simulink library "lat_dyn_haul_00"  (R2025a)
settings: Solver=VariableStepAuto  StartTime=0.0  StopTime=10.0  RelTol=1e-3
undefined symbols (not defined in the file): Cf, Cr, Lf, Lr, Machine_Mass, Payload
settings Model: Creator=marti343  LastModifiedBy=marti343

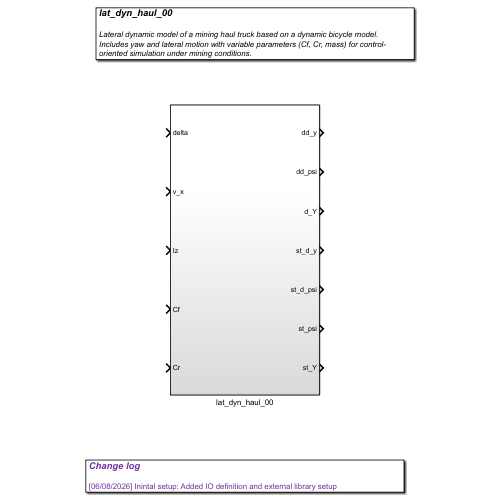
[thumbnail: Simulink's stored preview of the top-level diagram]
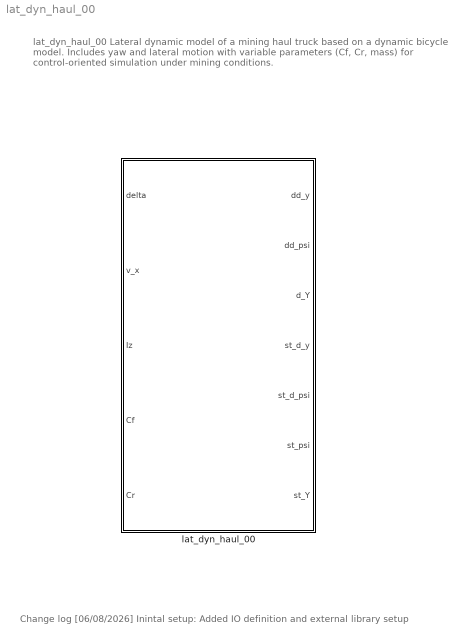
== system lat_dyn_haul_00 ==
  note: lat_dyn_haul_00
      |
      | Lateral dynamic model of a mining haul truck based on a dynamic bicycle model.
      | Includes yaw and lateral motion with variable parameters (Cf, Cr, mass) for control-oriented simulation under mining conditions.
  note: Change log
      |
      | [06/08/2026] Inintal setup: Added IO definition and external library setup
  lat_dyn_haul_00 : Subsystem

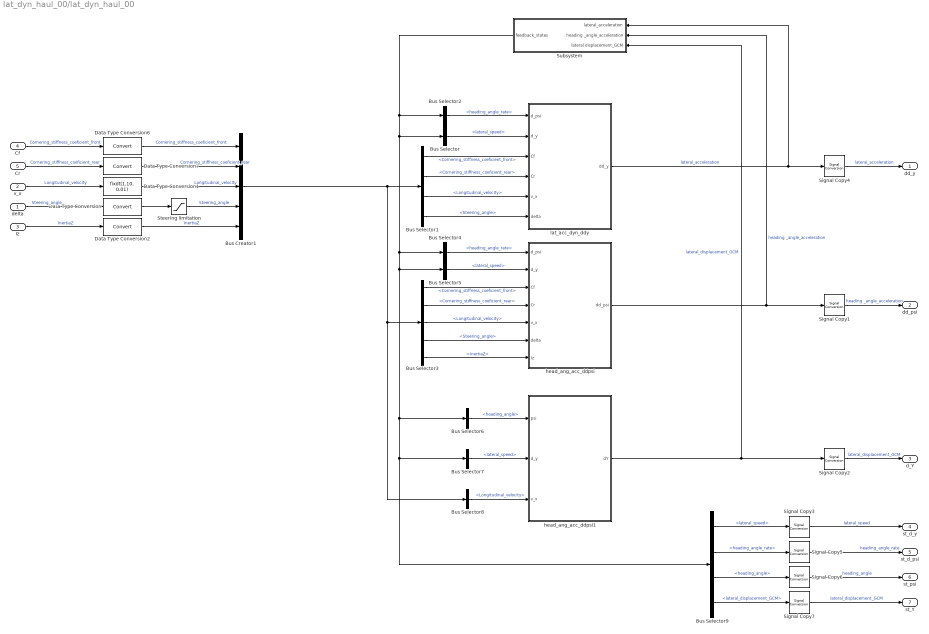
== system lat_dyn_haul_00/lat_dyn_haul_00 ==
  delta : Inport
  v_x : Inport  Port=2
  Iz : Inport  Port=3
  Cf : Inport  Port=4
  Cr : Inport  Port=5
  Bus Creator1 : BusCreator  Inputs=5
  Bus Selector : BusSelector  OutputSignals=lateral_speed
  Bus Selector1 : BusSelector  OutputSignals=Cornering_stiffness_coeficient_front,Cornering_stiffness_coeficient_rear,Longitudinal_velocity,Steering_angle
  Bus Selector2 : BusSelector  OutputSignals=heading_angle_rate
  Bus Selector3 : BusSelector  OutputSignals=Cornering_stiffness_coeficient_front,Cornering_stiffness_coeficient_rear,Longitudinal_velocity,Steering_angle,InertiaZ
  Bus Selector4 : BusSelector  OutputSignals=heading_angle_rate
  Bus Selector5 : BusSelector  OutputSignals=lateral_speed
  Bus Selector6 : BusSelector  OutputSignals=heading_angle
  Bus Selector7 : BusSelector  OutputSignals=lateral_speed
  Bus Selector8 : BusSelector  OutputSignals=Longitudinal_velocity
  Bus Selector9 : BusSelector  OutputSignals=lateral_speed,heading_angle_rate,heading_angle,lateral_displacement_GCM
  Data Type Conversion{,2,6..7} (4 alike) : DataTypeConversion  SaturateOnIntegerOverflow=off  RndMeth=Floor
  Data Type Conversion1 : DataTypeConversion  OutDataTypeStr=fixdt(1,10, 0.01)  SaturateOnIntegerOverflow=off  RndMeth=Floor
  Signal Copy{1..7} (7 alike) : SignalConversion  OverrideOpt=off
  Steering limitation : Saturate
  Subsystem : Subsystem
  head_ang_acc_ddpsi : Subsystem
  head_ang_acc_ddpsi1 : Subsystem
  lat_acc_dyn_ddy : Subsystem
  dd_y : Outport
  dd_psi : Outport  Port=2
  d_Y : Outport  Port=3
  st_d_y : Outport  Port=4
  st_d_psi : Outport  Port=5
  st_psi : Outport  Port=6
  st_Y : Outport  Port=7
  wires:
  delta/1 -> Data Type Conversion/1  "Steering_angle"
  Cf/1 -> Data Type Conversion6/1  "Cornering_stiffness_coeficient_front"
  Iz/1 -> Data Type Conversion2/1  "InertiaZ"
  v_x/1 -> Data Type Conversion1/1  "Longitudinal_velocity"
  Cr/1 -> Data Type Conversion7/1  "Cornering_stiffness_coeficient_rear"
  Data Type Conversion/1 -> Steering limitation/1
  Data Type Conversion6/1 -> Bus Creator1/1  "Cornering_stiffness_coeficient_front"
  Data Type Conversion7/1 -> Bus Creator1/2  "Cornering_stiffness_coeficient_rear"
  Data Type Conversion1/1 -> Bus Creator1/3  "Longitudinal_velocity"
  Steering limitation/1 -> Bus Creator1/4  "Steering_angle"
  lat_acc_dyn_ddy/1(dd_y) -> Subsystem/1(lateral_acceleration), Signal Copy4/1  "lateral_acceleration"
  Bus Selector/1 -> lat_acc_dyn_ddy/2(d_y)  "<lateral_speed>"
  Data Type Conversion2/1 -> Bus Creator1/5  "InertiaZ"
  Bus Creator1/1 -> Bus Selector8/1, Bus Selector3/1, Bus Selector1/1
  Bus Selector1/1 -> lat_acc_dyn_ddy/3(Cf)  "<Cornering_stiffness_coeficient_front>"
  Bus Selector1/2 -> lat_acc_dyn_ddy/4(Cr)  "<Cornering_stiffness_coeficient_rear>"
  Bus Selector1/3 -> lat_acc_dyn_ddy/5(v_x)  "<Longitudinal_velocity>"
  Bus Selector1/4 -> lat_acc_dyn_ddy/6(delta)  "<Steering_angle>"
  head_ang_acc_ddpsi/1(dd_psi) -> Subsystem/2(heading _angle_acceleration), Signal Copy1/1  "heading _angle_acceleration"
  Bus Selector2/1 -> lat_acc_dyn_ddy/1(d_psi)  "<heading_angle_rate>"
  Bus Selector3/1 -> head_ang_acc_ddpsi/3(Cf)  "<Cornering_stiffness_coeficient_front>"
  Bus Selector3/2 -> head_ang_acc_ddpsi/4(Cr)  "<Cornering_stiffness_coeficient_rear>"
  Bus Selector3/3 -> head_ang_acc_ddpsi/5(v_x)  "<Longitudinal_velocity>"
  Bus Selector3/4 -> head_ang_acc_ddpsi/6(delta)  "<Steering_angle>"
  Bus Selector3/5 -> head_ang_acc_ddpsi/7(Iz)  "<InertiaZ>"
  Bus Selector4/1 -> head_ang_acc_ddpsi/1(d_psi)  "<heading_angle_rate>"
  head_ang_acc_ddpsi1/1(dY) -> Subsystem/3(lateral displacement_GCM), Signal Copy2/1  "lateral_displacement_GCM"
  Bus Selector6/1 -> head_ang_acc_ddpsi1/1(psi)  "<heading_angle>"
  Bus Selector5/1 -> head_ang_acc_ddpsi/2(d_y)  "<lateral_speed>"
  Bus Selector7/1 -> head_ang_acc_ddpsi1/2(d_y)  "<lateral_speed>"
  Bus Selector8/1 -> head_ang_acc_ddpsi1/3(v_x)  "<Longitudinal_velocity>"
  Subsystem/1(feedback_states) -> Bus Selector2/1, Bus Selector9/1, Bus Selector7/1, Bus Selector6/1, Bus Selector5/1, Bus Selector4/1, Bus Selector/1
  Signal Copy4/1 -> dd_y/1  "lateral_acceleration"
  Signal Copy1/1 -> dd_psi/1  "heading _angle_acceleration"
  Signal Copy2/1 -> d_Y/1  "lateral_displacement_GCM"
  Bus Selector9/1 -> Signal Copy3/1  "<lateral_speed>"
  Bus Selector9/2 -> Signal Copy5/1  "<heading_angle_rate>"
  Bus Selector9/3 -> Signal Copy6/1  "<heading_angle>"
  Bus Selector9/4 -> Signal Copy7/1  "<lateral_displacement_GCM>"
  Signal Copy3/1 -> st_d_y/1  "lateral_speed"
  Signal Copy5/1 -> st_d_psi/1  "heading_angle_rate"
  Signal Copy6/1 -> st_psi/1  "heading_angle"
  Signal Copy7/1 -> st_Y/1  "lateral_displacement_GCM"

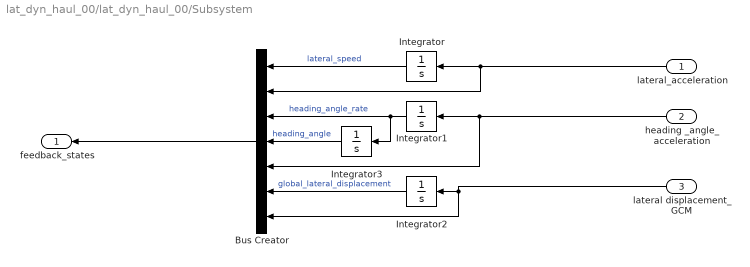
== system lat_dyn_haul_00/lat_dyn_haul_00/Subsystem ==
  lateral_acceleration : Inport
  heading _angle_acceleration : Inport  Port=2
  lateral displacement_GCM : Inport  Port=3
  Bus Creator : BusCreator  Inputs=7
  Integrator : Integrator
  Integrator1 : Integrator  InitialCondition=0.01
  Integrator2 : Integrator
  Integrator3 : Integrator
  feedback_states : Outport
  wires:
  Integrator1/1 -> Integrator3/1, Bus Creator/3  "heading_angle_rate"
  Integrator/1 -> Bus Creator/1  "lateral_speed"
  Integrator2/1 -> Bus Creator/6  "global_lateral_displacement"
  lateral_acceleration/1 -> Integrator/1, Bus Creator/2
  heading _angle_acceleration/1 -> Bus Creator/5, Integrator1/1
  lateral displacement_GCM/1 -> Bus Creator/7, Integrator2/1
  Integrator3/1 -> Bus Creator/4  "heading_angle"
  Bus Creator/1 -> feedback_states/1

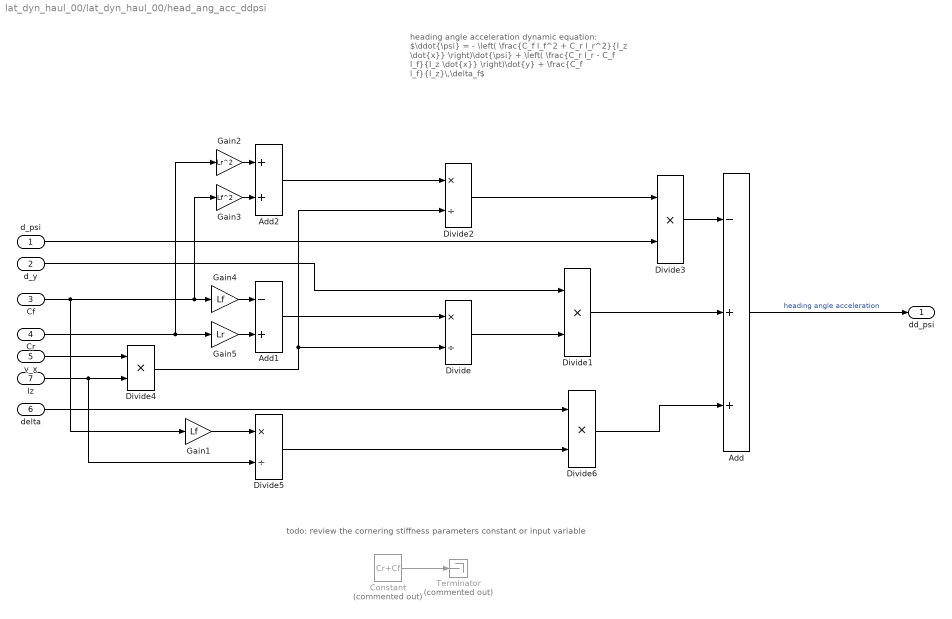
== system lat_dyn_haul_00/lat_dyn_haul_00/head_ang_acc_ddpsi ==
  note: heading angle acceleration dynamic equation:
      |
      | $\ddot{\psi} = - \left( \frac{C_f l_f^2 + C_r l_r^2}{I_z \dot{x}} \right)\dot{\psi} + \left( \frac{C_r l_r - C_f l_f}{I_z \dot{x}} \right)\dot{y} + \frac{C_f l_f}{I_z}\,\delta_f$
  note: todo: review the cornering stiffness parameters constant or input variable
  d_psi : Inport
  d_y : Inport  Port=2
  Cf : Inport  Port=3
  Cr : Inport  Port=4
  v_x : Inport  Port=5
  delta : Inport  Port=6
  Iz : Inport  Port=7
  Add : Sum  Inputs=-++
      settings: AttributesFormatString=|
      | Datatype = %<OutDataTypeStr>
      | Sample time = %<SampleTime>
  Add1 : Sum  Inputs=-+  OutDataTypeStr=double
      settings: AttributesFormatString=|
      | Datatype = %<OutDataTypeStr>
      | Sample time = %<SampleTime>
  Add2 : Sum  OutDataTypeStr=double
      settings: AttributesFormatString=|
      | Datatype = %<OutDataTypeStr>
      | Sample time = %<SampleTime>
  Constant : Constant  Commented=on  Value=Cr+Cf
  Divide : Product  Inputs=*/
      settings: AttributesFormatString=|
      | Datatype = %<OutDataTypeStr>
      | Sample time = %<SampleTime>
  Divide{1,3..4,6} (4 alike) : Product  Inputs=**
      Divide1 settings: AttributesFormatString=|
      | Datatype = %<OutDataTypeStr>
      | Sample time = %<SampleTime>
      Divide3 settings: AttributesFormatString=|
      | Datatype = %<OutDataTypeStr>
      | Sample time = %<SampleTime>
      Divide6 settings: AttributesFormatString=|
      | Datatype = %<OutDataTypeStr>
      | Sample time = %<SampleTime>
  Divide2 : Product  Inputs=*/
      settings: AttributesFormatString=|
      | Datatype = %<OutDataTypeStr>
      | Sample time = %<SampleTime>
  Divide5 : Product  Inputs=*/  OutDataTypeStr=double
      settings: AttributesFormatString=|
      | Datatype = %<OutDataTypeStr>
      | Sample time = %<SampleTime>
  Gain1 : Gain  Gain=Lf
  Gain2 : Gain  Gain=Lr^2
  Gain3 : Gain  Gain=Lf^2
  Gain4 : Gain  Gain=Lf
  Gain5 : Gain  Gain=Lr
  Terminator : Terminator  Commented=on
  dd_psi : Outport
  wires:
  d_psi/1 -> Divide3/2
  d_y/1 -> Divide1/1
  Divide6/1 -> Add/3
  Divide1/1 -> Add/2
  Divide2/1 -> Divide3/1
  Gain2/1 -> Add2/1
  Divide/1 -> Divide1/2
  Divide3/1 -> Add/1
  Add/1 -> dd_psi/1  "heading angle acceleration"
  delta/1 -> Divide6/1
  Cf/1 -> Gain1/1, Gain4/1, Gain3/1
  Constant/1 -> Terminator/1
  v_x/1 -> Divide4/1
  Divide4/1 -> Divide/2, Divide2/2
  Cr/1 -> Gain5/1, Gain2/1
  Gain3/1 -> Add2/2
  Add1/1 -> Divide/1
  Add2/1 -> Divide2/1
  Iz/1 -> Divide5/2, Divide4/2
  Gain4/1 -> Add1/1
  Gain5/1 -> Add1/2
  Gain1/1 -> Divide5/1
  Divide5/1 -> Divide6/2

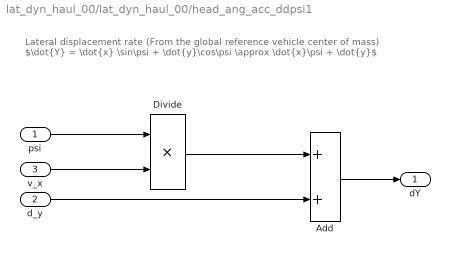
== system lat_dyn_haul_00/lat_dyn_haul_00/head_ang_acc_ddpsi1 ==
  note: Lateral displacement rate (From the global reference vehicle center of mass)
      | $\dot{Y} = \dot{x} \sin\psi + \dot{y}\cos\psi \approx \dot{x}\psi + \dot{y}$
  psi : Inport
  d_y : Inport  Port=2
  v_x : Inport  Port=3
  Add : Sum
  Divide : Product  Inputs=**
  dY : Outport
  wires:
  v_x/1 -> Divide/2
  psi/1 -> Divide/1
  Divide/1 -> Add/1
  d_y/1 -> Add/2
  Add/1 -> dY/1

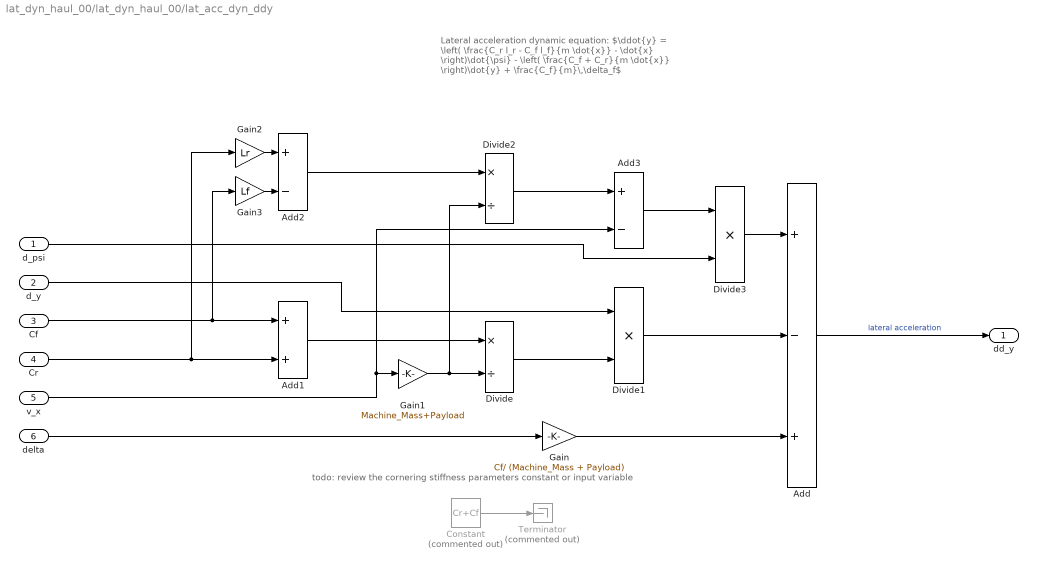
== system lat_dyn_haul_00/lat_dyn_haul_00/lat_acc_dyn_ddy ==
  note: todo: review the cornering stiffness parameters constant or input variable
  note: Lateral acceleration dynamic equation:
      |
      | $\ddot{y} = \left( \frac{C_r l_r - C_f l_f}{m \dot{x}} - \dot{x} \right)\dot{\psi} - \left( \frac{C_f + C_r}{m \dot{x}} \right)\dot{y} + \frac{C_f}{m}\,\delta_f$
  d_psi : Inport
  d_y : Inport  Port=2
  Cf : Inport  Port=3
  Cr : Inport  Port=4
  v_x : Inport  Port=5
  delta : Inport  Port=6
  Add : Sum  Inputs=+-+
      settings: AttributesFormatString=|
      | Datatype = %<OutDataTypeStr>
      | Sample time = %<SampleTime>
  Add1 : Sum  OutDataTypeStr=double
      settings: AttributesFormatString=|
      | Datatype = %<OutDataTypeStr>
      | Sample time = %<SampleTime>
  Add2 : Sum  Inputs=+-  OutDataTypeStr=double
      settings: AttributesFormatString=|
      | Datatype = %<OutDataTypeStr>
      | Sample time = %<SampleTime>
  Add3 : Sum  Inputs=+-
      settings: AttributesFormatString=|
      | Datatype = %<OutDataTypeStr>
      | Sample time = %<SampleTime>
  Constant : Constant  Commented=on  Value=Cr+Cf
  Divide : Product  Inputs=*/
      settings: AttributesFormatString=|
      | Datatype = %<OutDataTypeStr>
      | Sample time = %<SampleTime>
  Divide1 : Product  Inputs=**
      settings: AttributesFormatString=|
      | Datatype = %<OutDataTypeStr>
      | Sample time = %<SampleTime>
  Divide2 : Product  Inputs=*/
      settings: AttributesFormatString=|
      | Datatype = %<OutDataTypeStr>
      | Sample time = %<SampleTime>
  Divide3 : Product  Inputs=**
      settings: AttributesFormatString=|
      | Datatype = %<OutDataTypeStr>
      | Sample time = %<SampleTime>
  Gain : Gain  Gain=Cf/ (Machine_Mass + Payload)
  Gain1 : Gain  Gain=Machine_Mass+Payload
  Gain2 : Gain  Gain=Lr
  Gain3 : Gain  Gain=Lf
  Terminator : Terminator  Commented=on
  dd_y : Outport
  wires:
  Add2/1 -> Divide2/1
  Add1/1 -> Divide/1
  Gain3/1 -> Add2/2
  Cr/1 -> Gain2/1, Add1/2
  Gain1/1 -> Divide2/2, Divide/2
  v_x/1 -> Add3/2, Gain1/1
  Constant/1 -> Terminator/1
  Cf/1 -> Gain3/1, Add1/1
  delta/1 -> Gain/1
  Add/1 -> dd_y/1  "lateral acceleration"
  Divide3/1 -> Add/1
  Divide/1 -> Divide1/2
  Gain2/1 -> Add2/1
  Add3/1 -> Divide3/1
  Divide1/1 -> Add/2
  Divide2/1 -> Add3/1
  Gain/1 -> Add/3
  d_y/1 -> Divide1/1
  d_psi/1 -> Divide3/2
